simulink model "matrixOpsPractice"  (R2024b)
settings: Solver=VariableStepAuto  StartTime=0.0  StopTime=10.0  RelTol=1e-3
values from neighbouring files (symbols this model uses):
  C = [1  2  3; 4  5  6; 7  8  9]    [matrixOpsVar.mat]
  d = [1 2 4 5]    [matrixOpsVar.mat]
  m1 = [1  2; 3  4; 5  6]    [matrixOpsVar.mat]
  m2 = [1  1  1; 1  1  1]    [matrixOpsVar.mat]
  matrix_U = [0  1  2; 0  0  3; 0  0  4]    [matrixOpsVar.mat]
  SH = [0  2; -2  0]    [matrixOpsVar.mat]
  X = [1  2  3  4; 5  6  7  8; 9  10  11  21]    [matrixOpsVar.mat]
undefined symbols (not defined in the file or in its folder): gcbh, H1, Hermitian, Skew
libraries: matrix_library x7
settings Model: Creator=optimus  LastModifiedBy=optimus

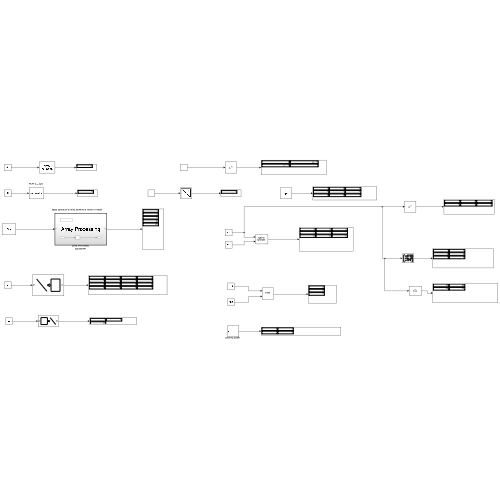
[thumbnail: Simulink's stored preview of the top-level diagram]
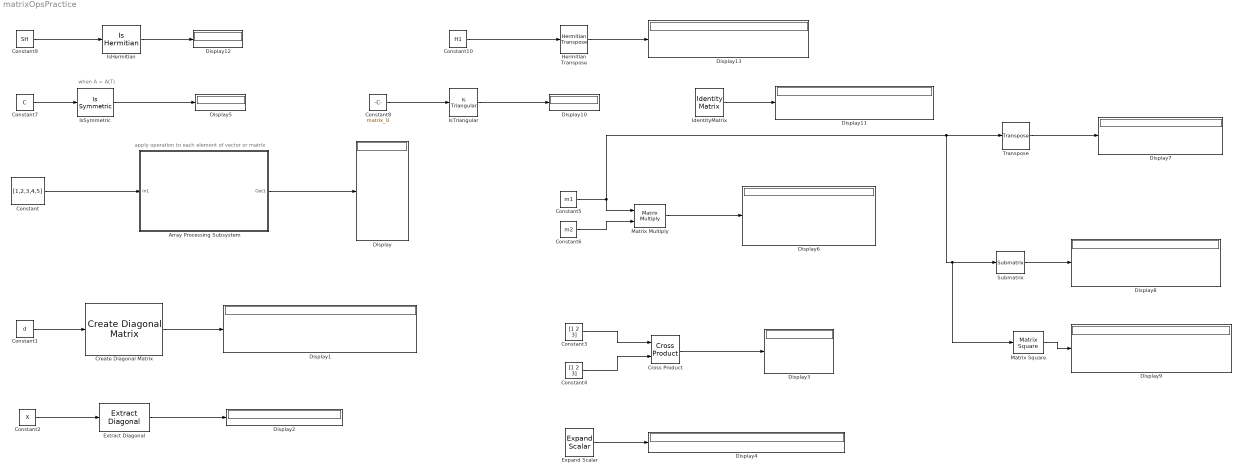
== system matrixOpsPractice ==
  note: when A = A(T)
  note: apply operation to each element of vector or matrix
  Array Processing Subsystem : Subsystem  ClipboardFcn=set_param(gcbh,'LinkStatus','breakWithoutHierarchy'); set_param(gcbh,'Mask','off'); set_param(gcbh,'MaskType',''); set_param(gcbh,'MaskDescription',''); set_param(gcbh,'OpenFcn',''); set_param(gcbh,'CopyFcn','')  TreatAsAtomicUnit=on
  Constant : Constant  Value=[1,2,3,4,5]
  Constant1 : Constant  Value=d
  Constant10 : Constant  Value=H1  VectorParams1D=off
  Constant2 : Constant  Value=X  VectorParams1D=off
  Constant3 : Constant  Value=[1 2 3]  VectorParams1D=off
  Constant4 : Constant  Value=[1 2 3]
  Constant5 : Constant  Value=m1
  Constant6 : Constant  Value=m2
  Constant7 : Constant  Value=C  VectorParams1D=off
  Constant8 : Constant  Value=matrix_U  VectorParams1D=off
  Constant9 : Constant  Value=SH  VectorParams1D=off
  Create Diagonal Matrix : matrix_library/Create Diagonal Matrix
      settings: LibrarySourceBlock=|
      | simulink/Matrix
      | Operations/Create Diagonal
      | Matrix
  Cross Product : matrix_library/Cross Product
  Display{,1..13} (14 alike) : Display
  Expand Scalar : ExpandScalar  OutputDimensions=[2 2]
  Extract Diagonal : matrix_library/Extract Diagonal
      settings: LibrarySourceBlock=|
      | simulink/Matrix
      | Operations/Extract Diagonal
  Hermitian Transpose : matrix_library/Hermitian Transpose
      settings: LibrarySourceBlock=|
      | simulink/Matrix
      | Operations/Hermitian Transpose
  IdentityMatrix : IdentityMatrix  OutputDimensions=3  OutDataTypeStr=uint8
  IsHermitian : IsHermitian  Mode=Skew-Hermitian
  IsSymmetric : IsSymmetric
  IsTriangular : IsTriangular
  Matrix Square : matrix_library/Matrix Square  OutMin=[]  OutMax=[]
      settings: LibrarySourceBlock=|
      | simulink/Matrix
      | Operations/Matrix
      | Square
  Matrix Multiply : Product  Multiplication=Matrix(*)
  Submatrix : matrix_library/Submatrix  RowSpan=All rows  RowStartMode=First  RowStartIndex=1  RowEndMode=Last  RowEndIndex=1  ColSpan=Range of columns  ColStartMode=First  ColStartIndex=1  ColEndMode=Offset from last  ColEndIndex=0
  Transpose : matrix_library/Transpose
  wires:
  Constant/1 -> Array Processing Subsystem/1(In1)
  Array Processing Subsystem/1(Out1) -> Display/1
  Create Diagonal Matrix/1 -> Display1/1
  Constant1/1 -> Create Diagonal Matrix/1
  Constant2/1 -> Extract Diagonal/1
  Extract Diagonal/1 -> Display2/1
  Cross Product/1 -> Display3/1
  Constant3/1 -> Cross Product/1
  Constant4/1 -> Cross Product/2
  Expand Scalar/1 -> Display4/1
  Matrix Multiply/1 -> Display6/1
  Transpose/1 -> Display7/1
  Submatrix/1 -> Display8/1
  Matrix Square/1 -> Display9/1
  Constant6/1 -> Matrix Multiply/2
  Constant5/1 -> Matrix Square/1, Submatrix/1, Transpose/1, Matrix Multiply/1
  IsSymmetric/1 -> Display5/1
  Constant7/1 -> IsSymmetric/1
  IsTriangular/1 -> Display10/1
  Constant8/1 -> IsTriangular/1
  IdentityMatrix/1 -> Display11/1
  IsHermitian/1 -> Display12/1
  Constant9/1 -> IsHermitian/1
  Hermitian Transpose/1 -> Display13/1
  Constant10/1 -> Hermitian Transpose/1

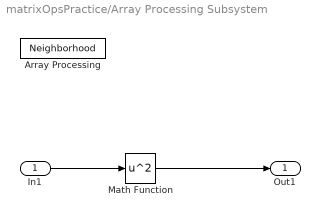
== system matrixOpsPractice/Array Processing Subsystem ==
  In1 : Inport
  Array Processing : Neighborhood  UsageType=ArrayFun
  Math Function : Math  Operator=square
  Out1 : Outport  ConcatenationDimension=[1 2]
  wires:
  In1/1 -> Math Function/1
  Math Function/1 -> Out1/1
